simulink model "Motor_Model_leadlag"  (R2022a)
settings: Solver=FixedStepAuto  StartTime=0.0  StopTime=inf  RelTol=1e-3
values from neighbouring files (symbols this model uses):
  b = 0.1    [main.m]
  J = 0.1    [main.m]
  K = 0.11    [main.m]
  L = 0.5    [main.m]
  R = 1    [main.m]
  Ts = 0.1    [main.m]
libraries: rllib x1
settings Model: Creator=sansh  LastModifiedBy=aizaQ
settings SolverCC: AlgebraicLoopSolver=TrustRegion
settings DebuggingCC: UnconnectedInputMsg=warning  UnconnectedOutputMsg=warning  UnconnectedLineMsg=warning  SFMachineParentedDataDiag=warning  ArithmeticOperatorsInVariantConditions=warning
settings SFSimCC: SimUseLocalCustomCode=off  CustomCodeUndefinedFunction=UseInterfaceOnly
settings RTWCC: RTWUseLocalCustomCode=off
settings CodeAppCC: StateflowObjectComments=on

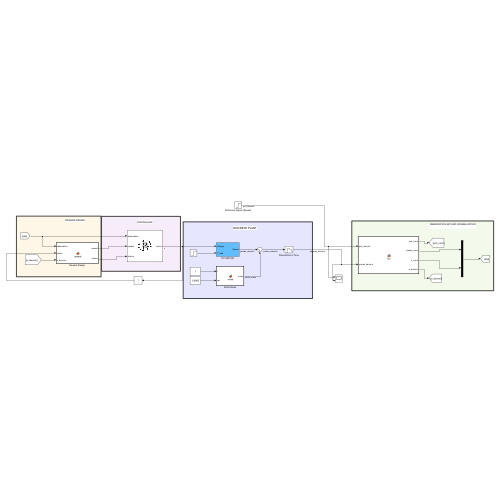
[thumbnail: Simulink's stored preview of the top-level diagram]
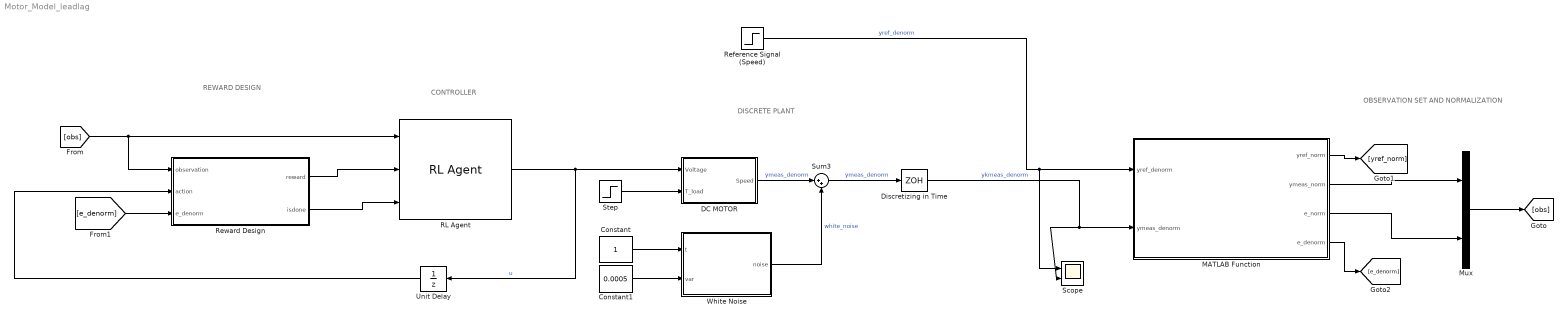
== system Motor_Model_leadlag ==
  note: REWARD DESIGN
  note: CONTROLLER
  note: OBSERVATION SET AND NORMALIZATION
  note: DISCRETE PLANT
  Constant : Constant  SampleTime=Ts
  Constant1 : Constant  Value=0.0005  SampleTime=Ts
  DC MOTOR : Subsystem
  Discretizing in Time : ZeroOrderHold  SampleTime=Ts
  MATLAB Function : MATLAB Function  TreatAsAtomicUnit=on
  Mux : Mux  Inputs=2
  RL Agent : rllib/RL Agent  Agent=agent  ExternalActionAsInput=off  ProvideLastAction=off  ProvideCumRwd=off  TreatAsDirectFeedthrough=on  UseStrictObservationDataTypes=off
  Reference Signal (Speed) : Step  Time=0  After=5  SampleTime=Ts
  Reward Design : MATLAB Function  TreatAsAtomicUnit=on
  Scope : Scope  NumInputPorts=2
  Step : Step  Time=0  After=0.001  SampleTime=Ts
  Sum3 : Sum  Inputs=|++
  Unit Delay : UnitDelay  SampleTime=Ts  HasFrameUpgradeWarning=on
  White Noise : MATLAB Function  TreatAsAtomicUnit=on
  wires:
  Reward Design/2(isdone) -> RL Agent/3
  Reward Design/1(reward) -> RL Agent/2
  RL Agent/1 -> Unit Delay/1, DC MOTOR/1(Voltage)  "u"
  DC MOTOR/1(Speed) -> Sum3/1  "ymeas_denorm"
  Constant/1 -> White Noise/1(t)
  White Noise/1(noise) -> Sum3/2  "white_noise"
  Constant1/1 -> White Noise/2(var)
  Unit Delay/1 -> Reward Design/2(action)
  Sum3/1 -> Discretizing in Time/1  "ymeas_denorm"
  Discretizing in Time/1 -> MATLAB Function/2(ymeas_denorm), Scope/2  "ykmeas_denorm"
  Step/1 -> DC MOTOR/2(T_load)
  Reference Signal (Speed)/1 -> Scope/1, MATLAB Function/1(yref_denorm)  "yref_denorm"
  Mux/1 -> [obs]
  [obs] -> Reward Design/1(observation), RL Agent/1
  MATLAB Function/3(e_norm) -> Mux/2
  MATLAB Function/2(ymeas_norm) -> Mux/1
  MATLAB Function/1(yref_norm) -> [yref_norm]
  MATLAB Function/4(e_denorm) -> [e_denorm]
  [e_denorm] -> Reward Design/3(e_denorm)

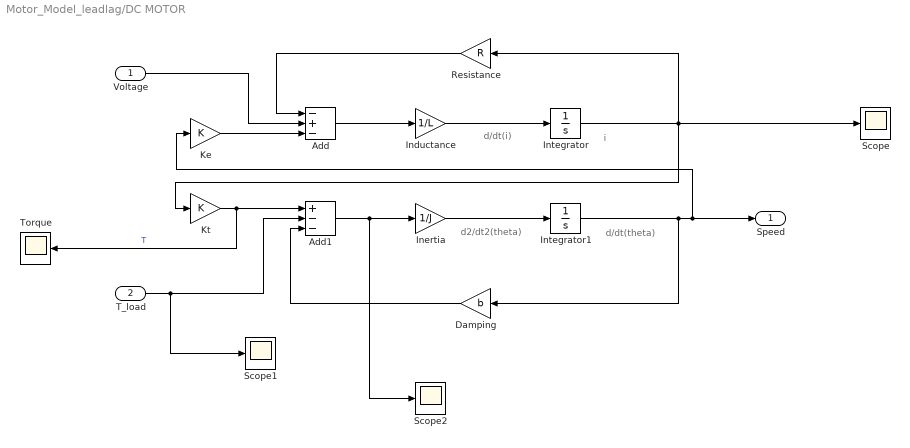
== system Motor_Model_leadlag/DC MOTOR ==
  note: i
  note: d/dt(i)
  note: d/dt(theta)
  note: d2/dt2(theta)
  Voltage : Inport
  T_load : Inport  Port=2
  Add : Sum  Inputs=-+-
  Add1 : Sum  Inputs=+--
  Damping : Gain  Gain=b
  Inductance : Gain  Gain=1/L
  Inertia : Gain  Gain=1/J
  Integrator : Integrator
  Integrator1 : Integrator
  Ke : Gain  Gain=K
  Kt : Gain  Gain=K
  Resistance : Gain  Gain=R
  Scope : Scope
  Scope1 : Scope
  Scope2 : Scope
  Torque : Scope
  Speed : Outport
  wires:
  Inductance/1 -> Integrator/1
  Integrator1/1 -> Damping/1, Speed/1, Ke/1
  Inertia/1 -> Integrator1/1
  Integrator/1 -> Scope/1, Resistance/1, Kt/1
  Kt/1 -> Torque/1, Add1/1  "T"
  Voltage/1 -> Add/2
  Resistance/1 -> Add/1
  Damping/1 -> Add1/3
  Ke/1 -> Add/3
  Add/1 -> Inductance/1
  Add1/1 -> Scope2/1, Inertia/1
  T_load/1 -> Scope1/1, Add1/2

== matlab function Motor_Model_leadlag/White Noise ==
  data: t input; noise output; var input
function noise  = noise(t,var)
    bruitn=rand(length(var),length(t));
    %bruitn=(bruit-(mean(bruit'))'*ones(1,length(t)))./((std(bruit'))'*ones(1,length(t)));
    noise=[(var(1)*bruitn(1,:)')];  
end

== matlab function Motor_Model_leadlag/Reward Design ==
  data: observation input; reward output; action input; isdone output; e_denorm input
function [reward,isdone] = reward(observation, action,e_denorm)


e = observation(2);
u = action;


Q = 2000;
R = 0.001;

% calculate reward value
reward = -(e_denorm'*Q*e_denorm)-(u'*R*u);

% done if succeeded the convergenze
% isdone = madeit
isdone = 0;

== matlab function Motor_Model_leadlag/MATLAB Function ==
  data: yref_norm output; ymeas_norm output; e_norm output; yref_denorm input; ymeas_denorm input; e_denorm output
function [yref_norm,ymeas_norm,e_norm,e_denorm] = fcn(yref_denorm,ymeas_denorm)

%% States NORMALIZATION

yref_max = 12;
yref_min = 0;

ymeas_max = 12;
ymeas_min = 0;


yref_norm = 2*((yref_denorm - yref_min)/(yref_max - yref_min)) - 1;

ymeas_norm = 2*((ymeas_denorm - ymeas_min)/(ymeas_max - ymeas_min)) - 1;


e_denorm = yref_denorm - ymeas_denorm;

e_max = 2;
e_min = -2;

e_norm = 2*((e_denorm - e_min)/(e_max - e_min)) - 1;
